simulink model "MBD_Switch"  (R2021b)
settings: Solver=FixedStepDiscrete  StartTime=0.0  StopTime=10.0  FixedStep=0.01  RelTol=1e-3
settings Model: Creator=waleed.elshemy  LastModifiedBy=waleed.elshemy

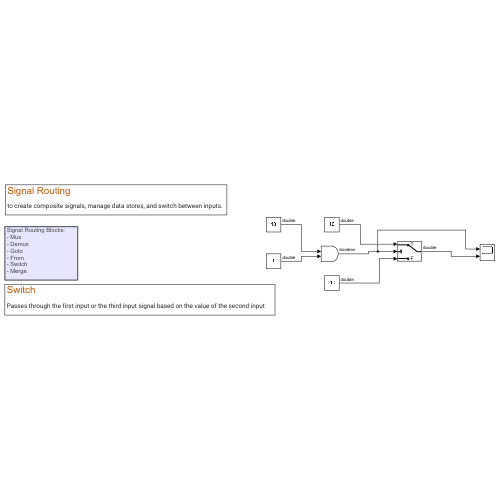
[thumbnail: Simulink's stored preview of the top-level diagram]
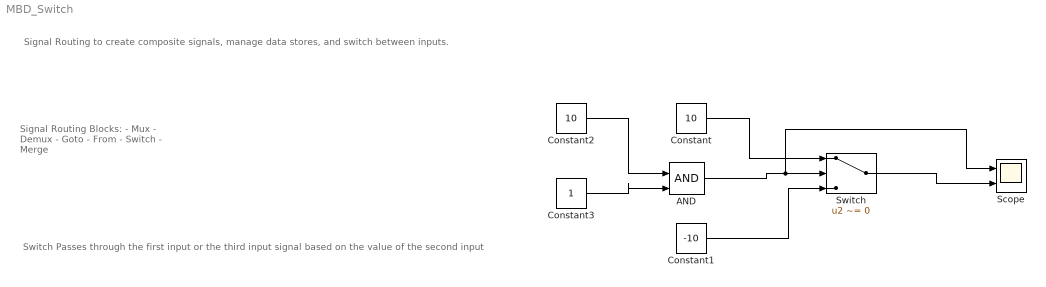
== system MBD_Switch ==
  note: Signal Routing
      | to create composite signals, manage data stores, and switch between inputs.
  note: Signal Routing Blocks:
      | - Mux
      | - Demux
      | - Goto
      | - From
      | - Switch
      | - Merge
  note: Switch
      | Passes through the first input or the third input signal based on the value of the second input
  AND : Logic  IconShape=distinctive  AllPortsSameDT=off  OutDataTypeStr=boolean
  Constant : Constant  Value=10
  Constant1 : Constant  Value=-10
  Constant2 : Constant  Value=10
  Constant3 : Constant
  Scope : Scope  NumInputPorts=2
  Switch : Switch  Criteria=u2 ~= 0  Threshold=3
  wires:
  Constant/1 -> Switch/1
  Constant1/1 -> Switch/3
  Switch/1 -> Scope/2
  AND/1 -> Scope/1, Switch/2
  Constant2/1 -> AND/1
  Constant3/1 -> AND/2
